simulink model "LQR_probleme_de_stabilizare"  (R2023b)
settings: Solver=VariableStepAuto  StartTime=0.0  StopTime=60  RelTol=1e-3
values from neighbouring files (symbols this model uses):
  A = [0 lambda 0 0 ... (first row only)    [rotary_inverted_pendulum.m]    (also in sis_liniar.m)
  B = [0; B21; 0; B41]./lambda    [rotary_inverted_pendulum.m]    (also in sis_liniar.m)
  K_fix = lqr(A,B,Q,R)    [rotary_inverted_pendulum.m]
settings Model: Creator=ovidiuceoca  LastModifiedBy=ovidiuceoca

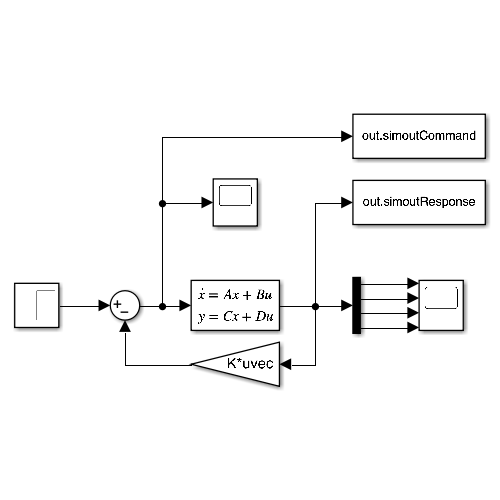
[thumbnail: Simulink's stored preview of the top-level diagram]
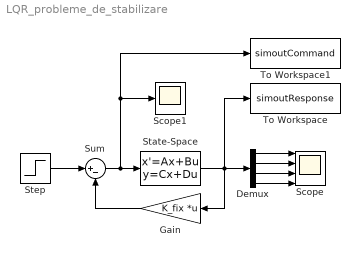
== system LQR_probleme_de_stabilizare ==
  Demux : Demux
  Gain : Gain  Gain=K_fix  Multiplication=Matrix(K*u) (u vector)
  Scope : Scope  NumInputPorts=4
  Scope1 : Scope
  State-Space : StateSpace  A=A  B=B  C=eye(4)  D=[0;0;0;0]  InitialCondition=[0; 0; 20; 0]
  Step : Step  Time=0  SampleTime=0
  Sum : Sum  Inputs=|+-
  To Workspace : ToWorkspace  VariableName=simoutResponse  SaveFormat=Timeseries  SampleTime=-1
  To Workspace1 : ToWorkspace  VariableName=simoutCommand  SaveFormat=Timeseries  SampleTime=-1
  wires:
  Sum/1 -> Scope1/1, To Workspace1/1, State-Space/1
  Gain/1 -> Sum/2
  Step/1 -> Sum/1
  State-Space/1 -> To Workspace/1, Gain/1, Demux/1
  Demux/4 -> Scope/4
  Demux/3 -> Scope/3
  Demux/2 -> Scope/2
  Demux/1 -> Scope/1
